simulink model "saturation"  (R2019a)
settings: Solver=VariableStepAuto  StartTime=0.0  StopTime=60  RelTol=1e-3
libraries: dspvision x1, simulink x1, dspobslib x1
settings Model: Creator=shse  LastModifiedBy=Ahmed

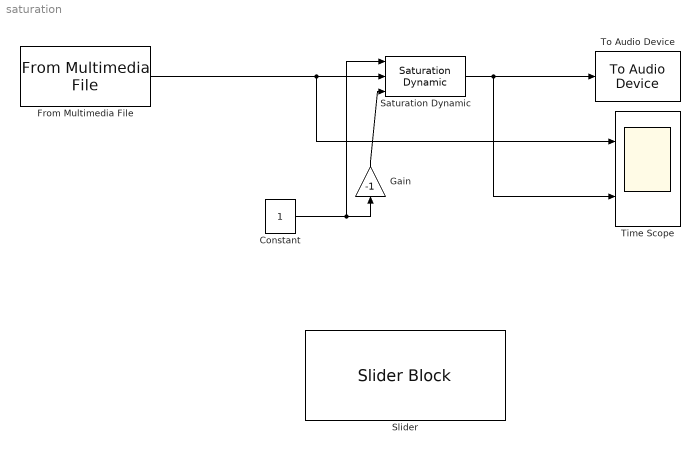
== system saturation ==
  Constant : Constant  VectorParams1D=off
  From Multimedia File : dspvision/From Multimedia File  inputFilename=C:\Users\Ahmed\Nextcloud\L3\LU3EE105\Audio\Documents de TP et projet-20191118\Projet\viv.wav  readRange=[1 Inf]  loop=on  numPlays=inf  outputStreams=Audio only  videoDataType=single  audioDataType=double  inheritSampleTime=on  userDefinedSampleTime=1/30  noAudioOutput=off  isIntensityVideo=off  fourcc=RGB  colorVideoFormat=Separate color signals  outputEOF=off  dataOrg=Column-major  audioFrameSize=1024  computeAudioFrameSize=off  outSamplingMode=Sample based
      settings: SourceProductName=DSP System Toolbox  SourceProductBaseCode=DS
  Gain : Gain  Gain=-1
  Saturation Dynamic : simulink/Discontinuities/Saturation Dynamic  OutMin=[]  OutMax=[]  OutDataTypeStr=Inherit: Same as second input  OutDataType=fixdt(1, 16)  OutScaling=2^-10  DoSatur=off
  Slider : SliderBlock  ScaleMax=1
  Time Scope : Scope  NumInputPorts=2
  To Audio Device : dspobslib/To Audio Device  deviceName=Default  inheritSampleRate=on  sampleRate=44100  deviceDatatype=Determine from input data type  autoBufferSize=on  bufferSize=4096  queueDuration=1.0  defaultOutputChannelMapping=on  outputChannelMapping=1:2  outputNumUnderrunSamples=off
      settings: SourceProductName=DSP System Toolbox  SourceProductBaseCode=DS
  wires:
  Gain/1 -> Saturation Dynamic/3
  Constant/1 -> Saturation Dynamic/1, Gain/1
  From Multimedia File/1 -> Time Scope/1, Saturation Dynamic/2
  Saturation Dynamic/1 -> Time Scope/2, To Audio Device/1
